simulink model "PID_Controller"  (R2020b)
settings: Solver=FixedStepAuto  StartTime=0.0  StopTime=120  RelTol=1e-3
values from neighbouring files (symbols this model uses):
  Kd = 0.49    [values.sldd]
  Ki = 4811.0    [values.sldd]
  Kp = 99.0    [values.sldd]
  n = 119827.0    [values.sldd]
settings Model: DataDictionary=values.sldd  Creator=shubham sharma  LastModifiedBy=shubham sharma
settings DataIOCC: SaveOutput=off  SaveTime=off

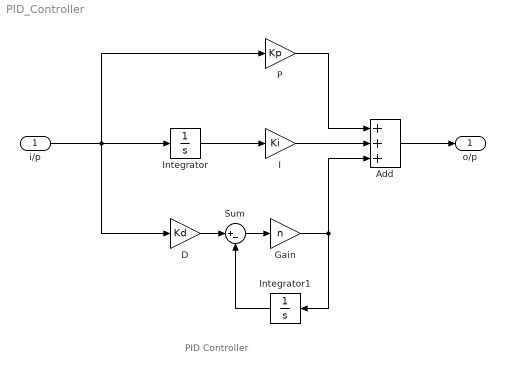
== system PID_Controller ==
  note: PID Controller
  i/p : Inport  OutDataTypeStr=double  PortDimensions=1  SampleTime=0
  Add : Sum  Inputs=+++
  D : Gain  Gain=Kd
  Gain : Gain  Gain=n
  I : Gain  Gain=Ki
  Integrator : Integrator
  Integrator1 : Integrator
  P : Gain  Gain=Kp
  Sum : Sum  Inputs=|+-
  o/p : Outport  OutDataTypeStr=double  PortDimensions=1  SampleTime=0
  wires:
  Integrator/1 -> I/1
  I/1 -> Add/2
  i/p/1 -> Integrator/1, P/1, D/1
  P/1 -> Add/1
  Add/1 -> o/p/1
  D/1 -> Sum/1
  Sum/1 -> Gain/1
  Gain/1 -> Integrator1/1, Add/3
  Integrator1/1 -> Sum/2
